simulink model "Multi_drones_deri_and_intro_compare"  (R2021a)
settings: Solver=ode4  StartTime=0.0  StopTime=50  FixedStep=0.005  RelTol=1e-3
(part 2 of 7)

== system Multi_drones_deri_and_intro_compare/Controller 4/High-level system ==
  L : Inport
  info_commu : Inport  Port=2
  bar_delta : Inport  Port=3
  a_d : Inport  Port=4
  Bus Creator : BusCreator  Inputs=3
  Bus Creator1 : BusCreator  Inputs=2
  Controller : MATLAB Function  TreatAsAtomicUnit=on
  Information subtracting : MATLAB Function  TreatAsAtomicUnit=on
  Saturation : Saturate  UpperLimit=0.2  LowerLimit=-0.2
  Virtual sliding variable 4 : Scope
  Virtual tracking error 4 : Scope
  bar_u_i : Scope
  bar_v : Integrator  InitialCondition=[0;0;0]  ContinuousStateAttributes='speed'
  bar_v_i : Scope
  bar_x : Integrator  Tag=Position_x1  InitialCondition=InitialCondition  ContinuousStateAttributes='position'
  bar_x_i : Scope
  new_ref : Outport
  States_virtual : Outport  Port=2
  wires:
  Information subtracting/1(delta_xi) -> Controller/1(delta_xi), Virtual tracking error 4/1
  Information subtracting/4(sat_dot) -> Controller/4(sat_dot)
  info_commu/1 -> Information subtracting/2(info_commu)
  bar_delta/1 -> Information subtracting/3(bar_delta)
  L/1 -> Information subtracting/1(L)
  a_d/1 -> Controller/5(a_di)
  bar_v/1 -> Bus Creator1/2, bar_v_i/1, Bus Creator/2, bar_x/1
  Bus Creator/1 -> new_ref/1
  bar_x/1 -> Bus Creator1/1, Bus Creator/1, bar_x_i/1
  Bus Creator1/1 -> States_virtual/1
  Controller/1(u_i) -> Saturation/1
  Saturation/1 -> bar_u_i/1, Bus Creator/3, bar_v/1
  Information subtracting/2(delta_vi) -> Controller/2(delta_vi)
  Information subtracting/3(s_i) -> Virtual sliding variable 4/1, Controller/3(s_i)

== system Multi_drones_deri_and_intro_compare/Controller 4/Quadcopter model ==
  u_i : Inport
  w_hat_p : Inport  Port=2
  w_hat_a : Inport  Port=3
  Add : Sum  Inputs=+-
  Add1 : Sum  Inputs=+-
  Bus Creator : BusCreator  Inputs=2
  Clock : Clock
  Quadcopter dynamics : MATLAB Function  TreatAsAtomicUnit=on
  f_a : Scope
  f_p : Scope
  quad_v : Scope
  quad_x : Scope
  v_int : Integrator  InitialCondition=[0;0;0;0;0;0]
  w_tilde_a : Scope
  w_tilde_p : Scope
  x_int : Integrator  InitialCondition=InitialCondition
  states_i : Outport
  wires:
  u_i/1 -> Quadcopter dynamics/2(u_i)
  Quadcopter dynamics/1(x_ddot) -> v_int/1
  x_int/1 -> Quadcopter dynamics/1(x_i), quad_x/1, Bus Creator/1
  v_int/1 -> Bus Creator/2, quad_v/1, Quadcopter dynamics/4(v_i), x_int/1
  Bus Creator/1 -> states_i/1
  Quadcopter dynamics/2(w_a) -> Add/1, f_a/1
  w_hat_a/1 -> Add/2
  Add/1 -> w_tilde_a/1
  Clock/1 -> Quadcopter dynamics/3(t)
  Quadcopter dynamics/3(w_p) -> f_p/1, Add1/1
  w_hat_p/1 -> Add1/2
  Add1/1 -> w_tilde_p/1

== system Multi_drones_deri_and_intro_compare/Controller 5/Controller ==
  note: Change the serial number here
  note: Change the serial number here
  note: Change the serial number here
  states_i : Inport
  ref_x_p : Inport  Port=2
  psi_id : Inport  Port=3
  Attitude controller : Subsystem
      settings: PortSchema="{\"entries\":[{\"content\":{\"sides\":[{\"content\":{\"connectorIds\":[\"In1\",\"In2\",\"In3\"]},\"type\":\"ConnectorPlacement.EquallySpacedRectSide\",\"uuid\":\"fa62b1eb-ed3d-4a84-b897-b51f17bb9d42\"},{\"content\":{\"connectorIds\":[\"Out1\"],\"side\":\"RIGHT\"},\"type\":\"ConnectorPlacement.EquallySpacedRectSide\",\"uuid\":\"9b6b7a3c-e484-45bf-bd32-fe40ffeb0d28\"},{\"content\":{\"connectorIds\":[\"Out2\"],\"side\":\"TOP\"},\"type\":\"ConnectorPlacement.EquallySpacedRectSide\",\"uuid\":\"d1ffdbb9-18c9-4f2c-95a6-bf4c2ab27347\"}]},\"type\":\"ConnectorPlacement.EquallySpacedConnector\",\"uuid\":\"2804a1df-60db-43d6-95d2-4687dde4bd06\"}],\"packageUris\":[\"http://schema.mathworks.com/mf0/Connector/R2020b\"],\"version\":\"1.0\"}"
  Constant : Constant  Value=13.72  VectorParams1D=off
  Manual Switch : ManualSwitch
  Nominal control calculation : MATLAB Function  TreatAsAtomicUnit=on
  Position controller1 : Subsystem
      settings: PortSchema="{\"entries\":[{\"content\":{\"sides\":[{\"content\":{\"connectorIds\":[\"In1\",\"In2\",\"In3\"]},\"type\":\"ConnectorPlacement.EquallySpacedRectSide\",\"uuid\":\"6f6db54a-065c-4c68-96d3-ce6f9528f7c2\"},{\"content\":{\"connectorIds\":[\"Out1\"],\"side\":\"RIGHT\"},\"type\":\"ConnectorPlacement.EquallySpacedRectSide\",\"uuid\":\"eab021de-0481-49e0-8239-dbc5993eb5fa\"},{\"content\":{\"connectorIds\":[\"Out2\"],\"side\":\"TOP\"},\"type\":\"ConnectorPlacement.EquallySpacedRectSide\",\"uuid\":\"c7d044cf-1b8b-40e5-8601-940ebebd0ccb\"},{\"content\":{\"connectorIds\":[],\"side\":\"BOTTOM\"},\"type\":\"ConnectorPlacement.EquallySpacedRectSide\",\"uuid\":\"6c5daa93-b438-4c34-9741-3ab1f6346320\"}]},\"type\":\"ConnectorPlacement.EquallySpacedConnector\",\"uuid\":\"bb7db914-9823-41d6-a8ba-39b4d2976335\"}],\"packageUris\":[\"http://schema.mathworks.com/mf0/Connector/R2020b\"],\"version\":\"1.0\"}"
  Real control input : MATLAB Function  TreatAsAtomicUnit=on
  Reverse calculation : Subsystem
      settings: PortSchema="{\"entries\":[{\"content\":{\"sides\":[{\"content\":{\"connectorIds\":[\"In1\",\"In2\"]},\"type\":\"ConnectorPlacement.EquallySpacedRectSide\",\"uuid\":\"a324fb00-881d-40c1-b7da-a9c7871d46ce\"},{\"content\":{\"connectorIds\":[\"Out1\",\"Out2\"],\"side\":\"RIGHT\"},\"type\":\"ConnectorPlacement.EquallySpacedRectSide\",\"uuid\":\"58739d0b-b2b3-44e8-8796-6553ce8d5a15\"},{\"content\":{\"connectorIds\":[\"In3\"],\"side\":\"TOP\"},\"type\":\"ConnectorPlacement.EquallySpacedRectSide\",\"uuid\":\"8c9acd48-a842-4889-b739-8799f04ac800\"}]},\"type\":\"ConnectorPlacement.EquallySpacedConnector\",\"uuid\":\"9c847f57-6425-42e5-8be7-b64809e08636\"}],\"packageUris\":[\"http://schema.mathworks.com/mf0/Connector/R2020b\"],\"version\":\"1.0\"}"
  Scope : Scope
  T_id : Scope
  atti_ref : Scope
  u : Scope
  u_ip : Scope
  u_nom_a : Scope
  u_nom_p : Scope
  u_i : Outport
  w_hat_p : Outport  Port=2
  w_hat_a : Outport  Port=3
  wires:
  Attitude controller/1(u_I_a) -> Real control input/1(u_i_a)
  ref_x_p/1 -> Position controller1/2(ref_x_p)
  states_i/1 -> Position controller1/1(states_i), Reverse calculation/3(states_i), Attitude controller/1(states_i), Nominal control calculation/1(states_i)
  Nominal control calculation/1(u_nom_p) -> Position controller1/3(u_nom_p), u_nom_p/1
  Nominal control calculation/2(u_nom_a) -> Attitude controller/3(u_nom_a), u_nom_a/1
  Position controller1/1(u_i_p) -> Reverse calculation/2(u_ip), u_ip/1
  Reverse calculation/1(atti_ref) -> Attitude controller/2(atti_ref), atti_ref/1
  Position controller1/2(w_hat_p) -> w_hat_p/1
  Attitude controller/2(w_hat_a) -> w_hat_a/1
  Constant/1 -> Manual Switch/2
  Reverse calculation/2(T_i_d) -> Manual Switch/1
  Manual Switch/1 -> T_id/1, Real control input/2(T_id)
  Real control input/2(u_i) -> Nominal control calculation/2(u_i), u/1, u_i/1
  Real control input/1(tau_i) -> Scope/1
  psi_id/1 -> Reverse calculation/1(psi_id)

== system Multi_drones_deri_and_intro_compare/Controller 5/High-level system ==
  L : Inport
  info_commu : Inport  Port=2
  bar_delta : Inport  Port=3
  a_d : Inport  Port=4
  Bus Creator : BusCreator  Inputs=3
  Bus Creator1 : BusCreator  Inputs=2
  Controller : MATLAB Function  TreatAsAtomicUnit=on
  Information subtracting : MATLAB Function  TreatAsAtomicUnit=on
  Saturation : Saturate  UpperLimit=0.2  LowerLimit=-0.2
  Virtual sliding variable 5 : Scope
  Virtual tracking error 5 : Scope
  bar_u_i : Scope
  bar_v : Integrator  InitialCondition=[0;0;0]  ContinuousStateAttributes='speed'
  bar_v_i : Scope
  bar_x : Integrator  Tag=Position_x1  InitialCondition=InitialCondition  ContinuousStateAttributes='position'
  bar_x_i : Scope
  new_ref : Outport
  States_virtual : Outport  Port=2
  wires:
  Information subtracting/1(delta_xi) -> Controller/1(delta_xi), Virtual tracking error 5/1
  Information subtracting/4(sat_dot) -> Controller/4(sat_dot)
  info_commu/1 -> Information subtracting/2(info_commu)
  bar_delta/1 -> Information subtracting/3(bar_delta)
  L/1 -> Information subtracting/1(L)
  a_d/1 -> Controller/5(a_di)
  bar_v/1 -> Bus Creator1/2, bar_v_i/1, Bus Creator/2, bar_x/1
  Bus Creator/1 -> new_ref/1
  bar_x/1 -> Bus Creator1/1, Bus Creator/1, bar_x_i/1
  Bus Creator1/1 -> States_virtual/1
  Controller/1(u_i) -> Saturation/1
  Saturation/1 -> bar_u_i/1, Bus Creator/3, bar_v/1
  Information subtracting/2(delta_vi) -> Controller/2(delta_vi)
  Information subtracting/3(s_i) -> Virtual sliding variable 5/1, Controller/3(s_i)

== system Multi_drones_deri_and_intro_compare/Controller 5/Quadcopter model ==
  u_i : Inport
  w_hat_p : Inport  Port=2
  w_hat_a : Inport  Port=3
  Add : Sum  Inputs=+-
  Add1 : Sum  Inputs=+-
  Bus Creator : BusCreator  Inputs=2
  Clock : Clock
  Quadcopter dynamics : MATLAB Function  TreatAsAtomicUnit=on
  f_a : Scope
  f_p : Scope
  quad_v : Scope
  quad_x : Scope
  v_int : Integrator  InitialCondition=[0;0;0;0;0;0]
  w_tilde_a : Scope
  w_tilde_p : Scope
  x_int : Integrator  InitialCondition=InitialCondition
  states_i : Outport
  wires:
  u_i/1 -> Quadcopter dynamics/2(u_i)
  Quadcopter dynamics/1(x_ddot) -> v_int/1
  x_int/1 -> Quadcopter dynamics/1(x_i), quad_x/1, Bus Creator/1
  v_int/1 -> Bus Creator/2, quad_v/1, Quadcopter dynamics/4(v_i), x_int/1
  Bus Creator/1 -> states_i/1
  Quadcopter dynamics/2(w_a) -> Add/1, f_a/1
  w_hat_a/1 -> Add/2
  Add/1 -> w_tilde_a/1
  Clock/1 -> Quadcopter dynamics/3(t)
  Quadcopter dynamics/3(w_p) -> f_p/1, Add1/1
  w_hat_p/1 -> Add1/2
  Add1/1 -> w_tilde_p/1

== system Multi_drones_deri_and_intro_compare/Controller 6/Controller ==
  note: Change the serial number here
  note: Change the serial number here
  note: Change the serial number here
  states_i : Inport
  ref_x_p : Inport  Port=2
  psi_id : Inport  Port=3
  Attitude controller : Subsystem
      settings: PortSchema="{\"entries\":[{\"content\":{\"sides\":[{\"content\":{\"connectorIds\":[\"In1\",\"In2\",\"In3\"]},\"type\":\"ConnectorPlacement.EquallySpacedRectSide\",\"uuid\":\"fa62b1eb-ed3d-4a84-b897-b51f17bb9d42\"},{\"content\":{\"connectorIds\":[\"Out1\"],\"side\":\"RIGHT\"},\"type\":\"ConnectorPlacement.EquallySpacedRectSide\",\"uuid\":\"9b6b7a3c-e484-45bf-bd32-fe40ffeb0d28\"},{\"content\":{\"connectorIds\":[\"Out2\"],\"side\":\"TOP\"},\"type\":\"ConnectorPlacement.EquallySpacedRectSide\",\"uuid\":\"d1ffdbb9-18c9-4f2c-95a6-bf4c2ab27347\"}]},\"type\":\"ConnectorPlacement.EquallySpacedConnector\",\"uuid\":\"2804a1df-60db-43d6-95d2-4687dde4bd06\"}],\"packageUris\":[\"http://schema.mathworks.com/mf0/Connector/R2020b\"],\"version\":\"1.0\"}"
  Constant : Constant  Value=13.72  VectorParams1D=off
  Manual Switch : ManualSwitch
  Nominal control calculation : MATLAB Function  TreatAsAtomicUnit=on
  Position controller1 : Subsystem
      settings: PortSchema="{\"entries\":[{\"content\":{\"sides\":[{\"content\":{\"connectorIds\":[\"In1\",\"In2\",\"In3\"]},\"type\":\"ConnectorPlacement.EquallySpacedRectSide\",\"uuid\":\"6f6db54a-065c-4c68-96d3-ce6f9528f7c2\"},{\"content\":{\"connectorIds\":[\"Out1\"],\"side\":\"RIGHT\"},\"type\":\"ConnectorPlacement.EquallySpacedRectSide\",\"uuid\":\"eab021de-0481-49e0-8239-dbc5993eb5fa\"},{\"content\":{\"connectorIds\":[\"Out2\"],\"side\":\"TOP\"},\"type\":\"ConnectorPlacement.EquallySpacedRectSide\",\"uuid\":\"c7d044cf-1b8b-40e5-8601-940ebebd0ccb\"},{\"content\":{\"connectorIds\":[],\"side\":\"BOTTOM\"},\"type\":\"ConnectorPlacement.EquallySpacedRectSide\",\"uuid\":\"6c5daa93-b438-4c34-9741-3ab1f6346320\"}]},\"type\":\"ConnectorPlacement.EquallySpacedConnector\",\"uuid\":\"bb7db914-9823-41d6-a8ba-39b4d2976335\"}],\"packageUris\":[\"http://schema.mathworks.com/mf0/Connector/R2020b\"],\"version\":\"1.0\"}"
  Real control input : MATLAB Function  TreatAsAtomicUnit=on
  Reverse calculation : Subsystem
      settings: PortSchema="{\"entries\":[{\"content\":{\"sides\":[{\"content\":{\"connectorIds\":[\"In1\",\"In2\"]},\"type\":\"ConnectorPlacement.EquallySpacedRectSide\",\"uuid\":\"a324fb00-881d-40c1-b7da-a9c7871d46ce\"},{\"content\":{\"connectorIds\":[\"Out1\",\"Out2\"],\"side\":\"RIGHT\"},\"type\":\"ConnectorPlacement.EquallySpacedRectSide\",\"uuid\":\"58739d0b-b2b3-44e8-8796-6553ce8d5a15\"},{\"content\":{\"connectorIds\":[\"In3\"],\"side\":\"TOP\"},\"type\":\"ConnectorPlacement.EquallySpacedRectSide\",\"uuid\":\"8c9acd48-a842-4889-b739-8799f04ac800\"}]},\"type\":\"ConnectorPlacement.EquallySpacedConnector\",\"uuid\":\"9c847f57-6425-42e5-8be7-b64809e08636\"}],\"packageUris\":[\"http://schema.mathworks.com/mf0/Connector/R2020b\"],\"version\":\"1.0\"}"
  Scope : Scope
  T_id : Scope
  atti_ref : Scope
  u : Scope
  u_ip : Scope
  u_nom_a : Scope
  u_nom_p : Scope
  u_i : Outport
  w_hat_p : Outport  Port=2
  w_hat_a : Outport  Port=3
  wires:
  Attitude controller/1(u_I_a) -> Real control input/1(u_i_a)
  ref_x_p/1 -> Position controller1/2(ref_x_p)
  states_i/1 -> Position controller1/1(states_i), Reverse calculation/3(states_i), Attitude controller/1(states_i), Nominal control calculation/1(states_i)
  Nominal control calculation/1(u_nom_p) -> Position controller1/3(u_nom_p), u_nom_p/1
  Nominal control calculation/2(u_nom_a) -> Attitude controller/3(u_nom_a), u_nom_a/1
  Position controller1/1(u_i_p) -> Reverse calculation/2(u_ip), u_ip/1
  Reverse calculation/1(atti_ref) -> Attitude controller/2(atti_ref), atti_ref/1
  Position controller1/2(w_hat_p) -> w_hat_p/1
  Attitude controller/2(w_hat_a) -> w_hat_a/1
  Constant/1 -> Manual Switch/2
  Reverse calculation/2(T_i_d) -> Manual Switch/1
  Manual Switch/1 -> T_id/1, Real control input/2(T_id)
  Real control input/2(u_i) -> Nominal control calculation/2(u_i), u/1, u_i/1
  Real control input/1(tau_i) -> Scope/1
  psi_id/1 -> Reverse calculation/1(psi_id)

== system Multi_drones_deri_and_intro_compare/Controller 6/High-level system ==
  L : Inport
  info_commu : Inport  Port=2
  bar_delta : Inport  Port=3
  a_d : Inport  Port=4
  Bus Creator : BusCreator  Inputs=3
  Bus Creator1 : BusCreator  Inputs=2
  Controller : MATLAB Function  TreatAsAtomicUnit=on
  Information subtracting : MATLAB Function  TreatAsAtomicUnit=on
  Saturation : Saturate  UpperLimit=0.2  LowerLimit=-0.2
  Virtual sliding variable : Scope
  Virtual tracking error : Scope
  bar_u_i : Scope
  bar_v : Integrator  InitialCondition=[0;0;0]  ContinuousStateAttributes='speed'
  bar_v_i : Scope
  bar_x : Integrator  Tag=Position_x1  InitialCondition=InitialCondition  ContinuousStateAttributes='position'
  bar_x_i : Scope
  new_ref : Outport
  States_virtual : Outport  Port=2
  wires:
  Information subtracting/1(delta_xi) -> Controller/1(delta_xi), Virtual tracking error/1
  Information subtracting/4(sat_dot) -> Controller/4(sat_dot)
  info_commu/1 -> Information subtracting/2(info_commu)
  bar_delta/1 -> Information subtracting/3(bar_delta)
  L/1 -> Information subtracting/1(L)
  a_d/1 -> Controller/5(a_di)
  bar_v/1 -> Bus Creator1/2, bar_v_i/1, Bus Creator/2, bar_x/1
  Bus Creator/1 -> new_ref/1
  bar_x/1 -> Bus Creator1/1, Bus Creator/1, bar_x_i/1
  Bus Creator1/1 -> States_virtual/1
  Controller/1(u_i) -> Saturation/1
  Saturation/1 -> bar_u_i/1, Bus Creator/3, bar_v/1
  Information subtracting/2(delta_vi) -> Controller/2(delta_vi)
  Information subtracting/3(s_i) -> Virtual sliding variable/1, Controller/3(s_i)

== system Multi_drones_deri_and_intro_compare/Controller 6/Quadcopter model ==
  u_i : Inport
  w_hat_p : Inport  Port=2
  w_hat_a : Inport  Port=3
  Add : Sum  Inputs=+-
  Add1 : Sum  Inputs=+-
  Bus Creator : BusCreator  Inputs=2
  Clock : Clock
  Quadcopter dynamics : MATLAB Function  TreatAsAtomicUnit=on
  f_a : Scope
  f_p : Scope
  quad_v : Scope
  quad_x : Scope
  v_int : Integrator  InitialCondition=[0;0;0;0;0;0]
  w_tilde_a : Scope
  w_tilde_p : Scope
  x_int : Integrator  InitialCondition=InitialCondition
  states_i : Outport
  wires:
  u_i/1 -> Quadcopter dynamics/2(u_i)
  Quadcopter dynamics/1(x_ddot) -> v_int/1
  x_int/1 -> Quadcopter dynamics/1(x_i), quad_x/1, Bus Creator/1
  v_int/1 -> Bus Creator/2, quad_v/1, Quadcopter dynamics/4(v_i), x_int/1
  Bus Creator/1 -> states_i/1
  Quadcopter dynamics/2(w_a) -> Add/1, f_a/1
  w_hat_a/1 -> Add/2
  Add/1 -> w_tilde_a/1
  Clock/1 -> Quadcopter dynamics/3(t)
  Quadcopter dynamics/3(w_p) -> f_p/1, Add1/1
  w_hat_p/1 -> Add1/2
  Add1/1 -> w_tilde_p/1

== system Multi_drones_deri_and_intro_compare/Reference generator/Coordinate reference ==
  Time : Inport
  Ref_gene : MATLAB Function  TreatAsAtomicUnit=on
  x_d_p : Outport
  v_d_p : Outport  Port=2
  a_d_p : Outport  Port=3
  wires:
  Time/1 -> Ref_gene/1(t)
  Ref_gene/1(x_d_p) -> x_d_p/1
  Ref_gene/2(v_d_p) -> v_d_p/1
  Ref_gene/3(a_d_p) -> a_d_p/1

== system Multi_drones_deri_and_intro_compare/Controller 1/Controller/Attitude controller ==
  states_i : Inport
  atti_ref : Inport  Port=2
  u_nom_a : Inport  Port=3
  Angle controller : MATLAB Function  TreatAsAtomicUnit=on
  Angle error : MATLAB Function  TreatAsAtomicUnit=on
  Angle sliding variable : MATLAB Function  TreatAsAtomicUnit=on
  Attitude loop observer : Subsystem
      settings: PortSchema="{\"entries\":[{\"content\":{\"sides\":[{\"content\":{\"connectorIds\":[\"In1\",\"In2\",\"In3\"]},\"type\":\"ConnectorPlacement.EquallySpacedRectSide\",\"uuid\":\"edf82c9f-eb15-4775-9311-d50d92fa47fd\"},{\"content\":{\"connectorIds\":[\"Out1\",\"Out2\"],\"side\":\"RIGHT\"},\"type\":\"ConnectorPlacement.EquallySpacedRectSide\",\"uuid\":\"b90416f6-8117-4ec7-8f9a-c5fae9711eab\"},{\"content\":{\"connectorIds\":[\"In4\"],\"side\":\"TOP\"},\"type\":\"ConnectorPlacement.EquallySpacedRectSide\",\"uuid\":\"e7e2e1a9-76d3-420a-917d-b73182cbe298\"}]},\"type\":\"ConnectorPlacement.EquallySpacedConnector\",\"uuid\":\"4fc8298e-c3da-4bdd-b1ba-c07bafbec956\"}],\"packageUris\":[\"http://schema.mathworks.com/mf0/Connector/R2020b\"],\"version\":\"1.0\"}"
  Scope : Scope
  Sliding mode differentiator : Subsystem
      settings: PortSchema="{\"entries\":[{\"content\":{\"sides\":[{\"content\":{\"connectorIds\":[\"In1\"]},\"type\":\"ConnectorPlacement.EquallySpacedRectSide\",\"uuid\":\"d0355641-aeac-4820-b7cd-f9621efbd127\"},{\"content\":{\"connectorIds\":[\"Out1\",\"Out2\"],\"side\":\"RIGHT\"},\"type\":\"ConnectorPlacement.EquallySpacedRectSide\",\"uuid\":\"185ec072-6206-4946-bebc-a6564ad10b6f\"},{\"content\":{\"connectorIds\":[\"Out3\"],\"side\":\"TOP\"},\"type\":\"ConnectorPlacement.EquallySpacedRectSide\",\"uuid\":\"43c1499b-0abd-4d60-8d0e-f99edfc99abb\"}]},\"type\":\"ConnectorPlacement.EquallySpacedConnector\",\"uuid\":\"7137f0d1-a693-433d-9f21-56f33280b1ef\"}],\"packageUris\":[\"http://schema.mathworks.com/mf0/Connector/R2020b\"],\"version\":\"1.0\"}"
  State selection : MATLAB Function  TreatAsAtomicUnit=on
  delta_v_a : Scope
  delta_x_a_1 : Scope
  s_i_a_1 : Scope
  u_I_a : Outport
  w_hat_a : Outport  Port=2
  wires:
  Angle controller/1(u_i_a) -> Scope/1, u_I_a/1
  Angle sliding variable/1(s_i_a) -> s_i_a_1/1, Angle controller/2(s_i_a)
  atti_ref/1 -> Sliding mode differentiator/1(Reference)
  states_i/1 -> State selection/1(states_i), Attitude loop observer/1(states_i)
  State selection/1(x_i_a) -> Attitude loop observer/2(x_i_a), Angle error/1(x_i_a)
  State selection/2(v_i_a) -> Attitude loop observer/3(v_i_a), Angle error/2(v_i_a)
  Sliding mode differentiator/3(ang_d) -> Angle error/3(ang_d)
  Angle error/1(delta_x_a) -> delta_x_a_1/1, Angle sliding variable/1(delta_x_a), Angle controller/3(delta_x_a)
  Angle error/2(delta_v_a) -> delta_v_a/1, Angle controller/4(delta_v_a), Angle sliding variable/2(delta_v_a)
  Attitude loop observer/2(w_hat_a) -> Angle controller/1(w_hat_a)
  Sliding mode differentiator/2(ang_d_ddot) -> Angle controller/5(ang_d_ddot)
  u_nom_a/1 -> Attitude loop observer/4(u_nom_a)
  Sliding mode differentiator/1(ang_d_dot) -> Angle error/4(ang_d_dot)
  Attitude loop observer/1(w_hat_a_actual) -> w_hat_a/1

== system Multi_drones_deri_and_intro_compare/Controller 1/Controller/Position controller1 ==
  note: Note that a saturation is added here
  states_i : Inport
  ref_x_p : Inport  Port=2
  u_nom_p : Inport  Port=3
  Constant : Constant  Value=[0;0;0]  VectorParams1D=off
  Error calculation : MATLAB Function  TreatAsAtomicUnit=on
  Position loop observer : Subsystem  mask{InitialCondition=[4;1;0]}
      mask prompts: InitialCondition "Simulink:blkprm_prompts:IntegratorInitCond"
      settings: PortSchema="{\"entries\":[{\"content\":{\"sides\":[{\"content\":{\"connectorIds\":[\"In1\",\"In2\",\"In3\"]},\"type\":\"ConnectorPlacement.EquallySpacedRectSide\",\"uuid\":\"edf82c9f-eb15-4775-9311-d50d92fa47fd\"},{\"content\":{\"connectorIds\":[\"Out1\",\"Out2\"],\"side\":\"RIGHT\"},\"type\":\"ConnectorPlacement.EquallySpacedRectSide\",\"uuid\":\"b90416f6-8117-4ec7-8f9a-c5fae9711eab\"},{\"content\":{\"connectorIds\":[\"In4\"],\"side\":\"TOP\"},\"type\":\"ConnectorPlacement.EquallySpacedRectSide\",\"uuid\":\"e7e2e1a9-76d3-420a-917d-b73182cbe298\"}]},\"type\":\"ConnectorPlacement.EquallySpacedConnector\",\"uuid\":\"4fc8298e-c3da-4bdd-b1ba-c07bafbec956\"}],\"packageUris\":[\"http://schema.mathworks.com/mf0/Connector/R2020b\"],\"version\":\"1.0\"}"
      mask TypeOptions InitialCondition: Integrator1/InitialCondition
      mask DialogControl InitialCondition Prompt: Initial condition:
  Reference selection (Low) : MATLAB Function  TreatAsAtomicUnit=on
  State selection : MATLAB Function  TreatAsAtomicUnit=on
  Virtual position controller : MATLAB Function  TreatAsAtomicUnit=on
  delta_v_p : Scope
  delta_x_p_1 : Scope
  s_i_p_1 : Scope
  u_i : Scope
  u_i_p : Outport
  w_hat_p : Outport  Port=2
  wires:
  states_i/1 -> Position loop observer/1(states_i), State selection/1(states_i)
  ref_x_p/1 -> Reference selection (Low)/1(ref_x_p)
  Reference selection (Low)/1(x_i_p_d) -> Error calculation/4(x_i_p_d)
  Reference selection (Low)/2(v_i_p_d) -> Error calculation/5(v_i_p_d)
  State selection/2(v_i_p) -> Position loop observer/3(v_i_p), Error calculation/2(v_i_p)
  State selection/1(x_i_p) -> Position loop observer/2(x_i_p), Error calculation/1(x_i_p)
  u_nom_p/1 -> Position loop observer/4(u_nom_p)
  Reference selection (Low)/3(a_i_p_d) -> Virtual position controller/5(a_i_p_d)
  Constant/1 -> Error calculation/3(Phi_i)
  Error calculation/3(delta_v_p) -> delta_v_p/1, Virtual position controller/4(delta_v_p)
  Error calculation/2(delta_x_p) -> delta_x_p_1/1, Virtual position controller/3(delta_x_p)
  Error calculation/1(s_i_p) -> s_i_p_1/1, Virtual position controller/2(s_i_p)
  Virtual position controller/1(u_i_p) -> u_i_p/1, u_i/1
  Position loop observer/1(w_hat_p_actual) -> w_hat_p/1
  Position loop observer/2(w_hat_p) -> Virtual position controller/1(w_hat_p)

== system Multi_drones_deri_and_intro_compare/Controller 1/Controller/Reverse calculation ==
  psi_id : Inport
  u_ip : Inport  Port=2
  states_i : Inport  Port=3
  Reverse calculation : MATLAB Function  TreatAsAtomicUnit=on
  State selection : MATLAB Function  TreatAsAtomicUnit=on
  atti_ref : Outport
  T_i_d : Outport  Port=2
  wires:
  Reverse calculation/2(T_i_d) -> T_i_d/1
  Reverse calculation/1(atti_ref) -> atti_ref/1
  states_i/1 -> State selection/1(states_i)
  State selection/1(x_i_a) -> Reverse calculation/3(x_i_a)
  u_ip/1 -> Reverse calculation/2(u_i_p)
  psi_id/1 -> Reverse calculation/1(psi_i_d)

== system Multi_drones_deri_and_intro_compare/Controller 2/Controller/Attitude controller ==
  states_i : Inport
  atti_ref : Inport  Port=2
  u_nom_a : Inport  Port=3
  Angle controller : MATLAB Function  TreatAsAtomicUnit=on
  Angle error : MATLAB Function  TreatAsAtomicUnit=on
  Angle sliding variable : MATLAB Function  TreatAsAtomicUnit=on
  Attitude loop observer : Subsystem
      settings: PortSchema="{\"entries\":[{\"content\":{\"sides\":[{\"content\":{\"connectorIds\":[\"In1\",\"In2\",\"In3\"]},\"type\":\"ConnectorPlacement.EquallySpacedRectSide\",\"uuid\":\"edf82c9f-eb15-4775-9311-d50d92fa47fd\"},{\"content\":{\"connectorIds\":[\"Out1\",\"Out2\"],\"side\":\"RIGHT\"},\"type\":\"ConnectorPlacement.EquallySpacedRectSide\",\"uuid\":\"b90416f6-8117-4ec7-8f9a-c5fae9711eab\"},{\"content\":{\"connectorIds\":[\"In4\"],\"side\":\"TOP\"},\"type\":\"ConnectorPlacement.EquallySpacedRectSide\",\"uuid\":\"e7e2e1a9-76d3-420a-917d-b73182cbe298\"}]},\"type\":\"ConnectorPlacement.EquallySpacedConnector\",\"uuid\":\"4fc8298e-c3da-4bdd-b1ba-c07bafbec956\"}],\"packageUris\":[\"http://schema.mathworks.com/mf0/Connector/R2020b\"],\"version\":\"1.0\"}"
  Scope : Scope
  Sliding mode differentiator : Subsystem
      settings: PortSchema="{\"entries\":[{\"content\":{\"sides\":[{\"content\":{\"connectorIds\":[\"In1\"]},\"type\":\"ConnectorPlacement.EquallySpacedRectSide\",\"uuid\":\"d0355641-aeac-4820-b7cd-f9621efbd127\"},{\"content\":{\"connectorIds\":[\"Out1\",\"Out2\"],\"side\":\"RIGHT\"},\"type\":\"ConnectorPlacement.EquallySpacedRectSide\",\"uuid\":\"185ec072-6206-4946-bebc-a6564ad10b6f\"},{\"content\":{\"connectorIds\":[\"Out3\"],\"side\":\"TOP\"},\"type\":\"ConnectorPlacement.EquallySpacedRectSide\",\"uuid\":\"43c1499b-0abd-4d60-8d0e-f99edfc99abb\"}]},\"type\":\"ConnectorPlacement.EquallySpacedConnector\",\"uuid\":\"7137f0d1-a693-433d-9f21-56f33280b1ef\"}],\"packageUris\":[\"http://schema.mathworks.com/mf0/Connector/R2020b\"],\"version\":\"1.0\"}"
  State selection : MATLAB Function  TreatAsAtomicUnit=on
  delta_v_a : Scope
  delta_x_a_2 : Scope
  s_i_a_2 : Scope
  u_I_a : Outport
  w_hat_a : Outport  Port=2
  wires:
  Angle controller/1(u_i_a) -> Scope/1, u_I_a/1
  Angle sliding variable/1(s_i_a) -> s_i_a_2/1, Angle controller/2(s_i_a)
  atti_ref/1 -> Sliding mode differentiator/1(Reference)
  states_i/1 -> State selection/1(states_i), Attitude loop observer/1(states_i)
  State selection/1(x_i_a) -> Attitude loop observer/2(x_i_a), Angle error/1(x_i_a)
  State selection/2(v_i_a) -> Attitude loop observer/3(v_i_a), Angle error/2(v_i_a)
  Sliding mode differentiator/3(ang_d) -> Angle error/3(ang_d)
  Angle error/1(delta_x_a) -> delta_x_a_2/1, Angle sliding variable/1(delta_x_a), Angle controller/3(delta_x_a)
  Angle error/2(delta_v_a) -> delta_v_a/1, Angle controller/4(delta_v_a), Angle sliding variable/2(delta_v_a)
  Attitude loop observer/2(w_hat_a) -> Angle controller/1(w_hat_a)
  Sliding mode differentiator/2(ang_d_ddot) -> Angle controller/5(ang_d_ddot)
  u_nom_a/1 -> Attitude loop observer/4(u_nom_a)
  Sliding mode differentiator/1(ang_d_dot) -> Angle error/4(ang_d_dot)
  Attitude loop observer/1(w_hat_a_actual) -> w_hat_a/1

== system Multi_drones_deri_and_intro_compare/Controller 2/Controller/Position controller1 ==
  note: Note that a saturation is added here
  states_i : Inport
  ref_x_p : Inport  Port=2
  u_nom_p : Inport  Port=3
  Constant : Constant  Value=[0;0;0]  VectorParams1D=off
  Error calculation : MATLAB Function  TreatAsAtomicUnit=on
  Position loop observer : Subsystem  mask{InitialCondition=[1;2;0]}
      mask prompts: InitialCondition "Simulink:blkprm_prompts:IntegratorInitCond"
      settings: PortSchema="{\"entries\":[{\"content\":{\"sides\":[{\"content\":{\"connectorIds\":[\"In1\",\"In2\",\"In3\"]},\"type\":\"ConnectorPlacement.EquallySpacedRectSide\",\"uuid\":\"edf82c9f-eb15-4775-9311-d50d92fa47fd\"},{\"content\":{\"connectorIds\":[\"Out1\",\"Out2\"],\"side\":\"RIGHT\"},\"type\":\"ConnectorPlacement.EquallySpacedRectSide\",\"uuid\":\"b90416f6-8117-4ec7-8f9a-c5fae9711eab\"},{\"content\":{\"connectorIds\":[\"In4\"],\"side\":\"TOP\"},\"type\":\"ConnectorPlacement.EquallySpacedRectSide\",\"uuid\":\"e7e2e1a9-76d3-420a-917d-b73182cbe298\"}]},\"type\":\"ConnectorPlacement.EquallySpacedConnector\",\"uuid\":\"4fc8298e-c3da-4bdd-b1ba-c07bafbec956\"}],\"packageUris\":[\"http://schema.mathworks.com/mf0/Connector/R2020b\"],\"version\":\"1.0\"}"
      mask TypeOptions InitialCondition: x_int/InitialCondition
      mask DialogControl InitialCondition Prompt: Initial condition:
  Reference selection (Low) : MATLAB Function  TreatAsAtomicUnit=on
  State selection : MATLAB Function  TreatAsAtomicUnit=on
  Virtual position controller : MATLAB Function  TreatAsAtomicUnit=on
  delta_v_p_2 : Scope
  delta_x_p_2 : Scope
  s_i_p_2 : Scope
  u_i : Scope
  u_i_p : Outport
  w_hat_p : Outport  Port=2
  wires:
  states_i/1 -> Position loop observer/1(states_i), State selection/1(states_i)
  ref_x_p/1 -> Reference selection (Low)/1(ref_x_p)
  Reference selection (Low)/1(x_i_p_d) -> Error calculation/4(x_i_p_d)
  Reference selection (Low)/2(v_i_p_d) -> Error calculation/5(v_i_p_d)
  State selection/2(v_i_p) -> Position loop observer/3(v_i_p), Error calculation/2(v_i_p)
  State selection/1(x_i_p) -> Position loop observer/2(x_i_p), Error calculation/1(x_i_p)
  u_nom_p/1 -> Position loop observer/4(u_nom_p)
  Position loop observer/2(w_hat_p) -> Virtual position controller/1(w_hat_p)
  Reference selection (Low)/3(a_i_p_d) -> Virtual position controller/5(a_i_p_d)
  Constant/1 -> Error calculation/3(Phi_i)
  Error calculation/3(delta_v_p) -> delta_v_p_2/1, Virtual position controller/4(delta_v_p)
  Error calculation/2(delta_x_p) -> delta_x_p_2/1, Virtual position controller/3(delta_x_p)
  Error calculation/1(s_i_p) -> s_i_p_2/1, Virtual position controller/2(s_i_p)
  Virtual position controller/1(u_i_p) -> u_i_p/1, u_i/1
  Position loop observer/1(w_hat_p_actual) -> w_hat_p/1

== system Multi_drones_deri_and_intro_compare/Controller 2/Controller/Reverse calculation ==
  psi_id : Inport
  u_ip : Inport  Port=2
  states_i : Inport  Port=3
  Reverse calculation : MATLAB Function  TreatAsAtomicUnit=on
  State selection : MATLAB Function  TreatAsAtomicUnit=on
  atti_ref : Outport
  T_i_d : Outport  Port=2
  wires:
  Reverse calculation/2(T_i_d) -> T_i_d/1
  Reverse calculation/1(atti_ref) -> atti_ref/1
  states_i/1 -> State selection/1(states_i)
  State selection/1(x_i_a) -> Reverse calculation/3(x_i_a)
  u_ip/1 -> Reverse calculation/2(u_i_p)
  psi_id/1 -> Reverse calculation/1(psi_i_d)

== system Multi_drones_deri_and_intro_compare/Controller 3/Controller/Attitude controller ==
  states_i : Inport
  atti_ref : Inport  Port=2
  u_nom_a : Inport  Port=3
  Angle controller : MATLAB Function  TreatAsAtomicUnit=on
  Angle error : MATLAB Function  TreatAsAtomicUnit=on
  Angle sliding variable : MATLAB Function  TreatAsAtomicUnit=on
  Attitude loop observer : Subsystem
      settings: PortSchema="{\"entries\":[{\"content\":{\"sides\":[{\"content\":{\"connectorIds\":[\"In1\",\"In2\",\"In3\"]},\"type\":\"ConnectorPlacement.EquallySpacedRectSide\",\"uuid\":\"edf82c9f-eb15-4775-9311-d50d92fa47fd\"},{\"content\":{\"connectorIds\":[\"Out1\",\"Out2\"],\"side\":\"RIGHT\"},\"type\":\"ConnectorPlacement.EquallySpacedRectSide\",\"uuid\":\"b90416f6-8117-4ec7-8f9a-c5fae9711eab\"},{\"content\":{\"connectorIds\":[\"In4\"],\"side\":\"TOP\"},\"type\":\"ConnectorPlacement.EquallySpacedRectSide\",\"uuid\":\"e7e2e1a9-76d3-420a-917d-b73182cbe298\"}]},\"type\":\"ConnectorPlacement.EquallySpacedConnector\",\"uuid\":\"4fc8298e-c3da-4bdd-b1ba-c07bafbec956\"}],\"packageUris\":[\"http://schema.mathworks.com/mf0/Connector/R2020b\"],\"version\":\"1.0\"}"
  Scope : Scope
  Sliding mode differentiator : Subsystem
      settings: PortSchema="{\"entries\":[{\"content\":{\"sides\":[{\"content\":{\"connectorIds\":[\"In1\"]},\"type\":\"ConnectorPlacement.EquallySpacedRectSide\",\"uuid\":\"d0355641-aeac-4820-b7cd-f9621efbd127\"},{\"content\":{\"connectorIds\":[\"Out1\",\"Out2\"],\"side\":\"RIGHT\"},\"type\":\"ConnectorPlacement.EquallySpacedRectSide\",\"uuid\":\"185ec072-6206-4946-bebc-a6564ad10b6f\"},{\"content\":{\"connectorIds\":[\"Out3\"],\"side\":\"TOP\"},\"type\":\"ConnectorPlacement.EquallySpacedRectSide\",\"uuid\":\"43c1499b-0abd-4d60-8d0e-f99edfc99abb\"}]},\"type\":\"ConnectorPlacement.EquallySpacedConnector\",\"uuid\":\"7137f0d1-a693-433d-9f21-56f33280b1ef\"}],\"packageUris\":[\"http://schema.mathworks.com/mf0/Connector/R2020b\"],\"version\":\"1.0\"}"
  State selection : MATLAB Function  TreatAsAtomicUnit=on
  delta_v_a : Scope
  delta_x_a_3 : Scope
  s_i_a_3 : Scope
  u_I_a : Outport
  w_hat_a : Outport  Port=2
  wires:
  Angle controller/1(u_i_a) -> Scope/1, u_I_a/1
  Angle sliding variable/1(s_i_a) -> s_i_a_3/1, Angle controller/2(s_i_a)
  atti_ref/1 -> Sliding mode differentiator/1(Reference)
  states_i/1 -> State selection/1(states_i), Attitude loop observer/1(states_i)
  State selection/1(x_i_a) -> Attitude loop observer/2(x_i_a), Angle error/1(x_i_a)
  State selection/2(v_i_a) -> Attitude loop observer/3(v_i_a), Angle error/2(v_i_a)
  Sliding mode differentiator/3(ang_d) -> Angle error/3(ang_d)
  Angle error/1(delta_x_a) -> delta_x_a_3/1, Angle sliding variable/1(delta_x_a), Angle controller/3(delta_x_a)
  Angle error/2(delta_v_a) -> delta_v_a/1, Angle controller/4(delta_v_a), Angle sliding variable/2(delta_v_a)
  Attitude loop observer/2(w_hat_a) -> Angle controller/1(w_hat_a)
  Sliding mode differentiator/2(ang_d_ddot) -> Angle controller/5(ang_d_ddot)
  u_nom_a/1 -> Attitude loop observer/4(u_nom_a)
  Sliding mode differentiator/1(ang_d_dot) -> Angle error/4(ang_d_dot)
  Attitude loop observer/1(w_hat_a_actual) -> w_hat_a/1

== system Multi_drones_deri_and_intro_compare/Controller 3/Controller/Position controller1 ==
  states_i : Inport
  ref_x_p : Inport  Port=2
  u_nom_p : Inport  Port=3
  Constant : Constant  Value=[0;0;0]  VectorParams1D=off
  Error calculation : MATLAB Function  TreatAsAtomicUnit=on
  Position loop observer : Subsystem  mask{InitialCondition=[-2;4;0]}
      mask prompts: InitialCondition "Simulink:blkprm_prompts:IntegratorInitCond"
      settings: PortSchema="{\"entries\":[{\"content\":{\"sides\":[{\"content\":{\"connectorIds\":[\"In1\",\"In2\",\"In3\"]},\"type\":\"ConnectorPlacement.EquallySpacedRectSide\",\"uuid\":\"edf82c9f-eb15-4775-9311-d50d92fa47fd\"},{\"content\":{\"connectorIds\":[\"Out1\",\"Out2\"],\"side\":\"RIGHT\"},\"type\":\"ConnectorPlacement.EquallySpacedRectSide\",\"uuid\":\"b90416f6-8117-4ec7-8f9a-c5fae9711eab\"},{\"content\":{\"connectorIds\":[\"In4\"],\"side\":\"TOP\"},\"type\":\"ConnectorPlacement.EquallySpacedRectSide\",\"uuid\":\"e7e2e1a9-76d3-420a-917d-b73182cbe298\"}]},\"type\":\"ConnectorPlacement.EquallySpacedConnector\",\"uuid\":\"4fc8298e-c3da-4bdd-b1ba-c07bafbec956\"}],\"packageUris\":[\"http://schema.mathworks.com/mf0/Connector/R2020b\"],\"version\":\"1.0\"}"
      mask TypeOptions InitialCondition: x_int/InitialCondition
      mask DialogControl InitialCondition Prompt: Initial condition:
  Reference selection (Low) : MATLAB Function  TreatAsAtomicUnit=on
  State selection : MATLAB Function  TreatAsAtomicUnit=on
  Virtual position controller : MATLAB Function  TreatAsAtomicUnit=on
  delta_v_p_2 : Scope
  delta_x_p_3 : Scope
  s_i_p_3 : Scope
  u_i : Scope
  u_i_p : Outport
  w_hat_p : Outport  Port=2
  wires:
  states_i/1 -> Position loop observer/1(states_i), State selection/1(states_i)
  ref_x_p/1 -> Reference selection (Low)/1(ref_x_p)
  Reference selection (Low)/1(x_i_p_d) -> Error calculation/4(x_i_p_d)
  Reference selection (Low)/2(v_i_p_d) -> Error calculation/5(v_i_p_d)
  State selection/2(v_i_p) -> Position loop observer/3(v_i_p), Error calculation/2(v_i_p)
  State selection/1(x_i_p) -> Position loop observer/2(x_i_p), Error calculation/1(x_i_p)
  u_nom_p/1 -> Position loop observer/4(u_nom_p)
  Position loop observer/2(w_hat_p) -> Virtual position controller/1(w_hat_p)
  Reference selection (Low)/3(a_i_p_d) -> Virtual position controller/5(a_i_p_d)
  Constant/1 -> Error calculation/3(Phi_i)
  Error calculation/3(delta_v_p) -> delta_v_p_2/1, Virtual position controller/4(delta_v_p)
  Error calculation/2(delta_x_p) -> delta_x_p_3/1, Virtual position controller/3(delta_x_p)
  Error calculation/1(s_i_p) -> s_i_p_3/1, Virtual position controller/2(s_i_p)
  Virtual position controller/1(u_i_p) -> u_i_p/1, u_i/1
  Position loop observer/1(w_hat_p_actual) -> w_hat_p/1

== system Multi_drones_deri_and_intro_compare/Controller 3/Controller/Reverse calculation ==
  psi_id : Inport
  u_ip : Inport  Port=2
  states_i : Inport  Port=3
  Reverse calculation : MATLAB Function  TreatAsAtomicUnit=on
  State selection : MATLAB Function  TreatAsAtomicUnit=on
  atti_ref : Outport
  T_i_d : Outport  Port=2
  wires:
  Reverse calculation/2(T_i_d) -> T_i_d/1
  Reverse calculation/1(atti_ref) -> atti_ref/1
  states_i/1 -> State selection/1(states_i)
  State selection/1(x_i_a) -> Reverse calculation/3(x_i_a)
  u_ip/1 -> Reverse calculation/2(u_i_p)
  psi_id/1 -> Reverse calculation/1(psi_i_d)

== system Multi_drones_deri_and_intro_compare/Controller 4/Controller/Attitude controller ==
  states_i : Inport
  atti_ref : Inport  Port=2
  u_nom_a : Inport  Port=3
  Angle controller : MATLAB Function  TreatAsAtomicUnit=on
  Angle error : MATLAB Function  TreatAsAtomicUnit=on
  Angle sliding variable : MATLAB Function  TreatAsAtomicUnit=on
  Attitude loop observer : Subsystem
      settings: PortSchema="{\"entries\":[{\"content\":{\"sides\":[{\"content\":{\"connectorIds\":[\"In1\",\"In2\",\"In3\"]},\"type\":\"ConnectorPlacement.EquallySpacedRectSide\",\"uuid\":\"edf82c9f-eb15-4775-9311-d50d92fa47fd\"},{\"content\":{\"connectorIds\":[\"Out1\",\"Out2\"],\"side\":\"RIGHT\"},\"type\":\"ConnectorPlacement.EquallySpacedRectSide\",\"uuid\":\"b90416f6-8117-4ec7-8f9a-c5fae9711eab\"},{\"content\":{\"connectorIds\":[\"In4\"],\"side\":\"TOP\"},\"type\":\"ConnectorPlacement.EquallySpacedRectSide\",\"uuid\":\"e7e2e1a9-76d3-420a-917d-b73182cbe298\"}]},\"type\":\"ConnectorPlacement.EquallySpacedConnector\",\"uuid\":\"4fc8298e-c3da-4bdd-b1ba-c07bafbec956\"}],\"packageUris\":[\"http://schema.mathworks.com/mf0/Connector/R2020b\"],\"version\":\"1.0\"}"
  Scope : Scope
  Sliding mode differentiator : Subsystem
      settings: PortSchema="{\"entries\":[{\"content\":{\"sides\":[{\"content\":{\"connectorIds\":[\"In1\"]},\"type\":\"ConnectorPlacement.EquallySpacedRectSide\",\"uuid\":\"d0355641-aeac-4820-b7cd-f9621efbd127\"},{\"content\":{\"connectorIds\":[\"Out1\",\"Out2\"],\"side\":\"RIGHT\"},\"type\":\"ConnectorPlacement.EquallySpacedRectSide\",\"uuid\":\"185ec072-6206-4946-bebc-a6564ad10b6f\"},{\"content\":{\"connectorIds\":[\"Out3\"],\"side\":\"TOP\"},\"type\":\"ConnectorPlacement.EquallySpacedRectSide\",\"uuid\":\"43c1499b-0abd-4d60-8d0e-f99edfc99abb\"}]},\"type\":\"ConnectorPlacement.EquallySpacedConnector\",\"uuid\":\"7137f0d1-a693-433d-9f21-56f33280b1ef\"}],\"packageUris\":[\"http://schema.mathworks.com/mf0/Connector/R2020b\"],\"version\":\"1.0\"}"
  State selection : MATLAB Function  TreatAsAtomicUnit=on
  delta_v_a : Scope
  delta_x_a_4 : Scope
  s_i_a_4 : Scope
  u_I_a : Outport
  w_hat_a : Outport  Port=2
  wires:
  Angle controller/1(u_i_a) -> Scope/1, u_I_a/1
  Angle sliding variable/1(s_i_a) -> s_i_a_4/1, Angle controller/2(s_i_a)
  atti_ref/1 -> Sliding mode differentiator/1(Reference)
  states_i/1 -> State selection/1(states_i), Attitude loop observer/1(states_i)
  State selection/1(x_i_a) -> Attitude loop observer/2(x_i_a), Angle error/1(x_i_a)
  State selection/2(v_i_a) -> Attitude loop observer/3(v_i_a), Angle error/2(v_i_a)
  Sliding mode differentiator/3(ang_d) -> Angle error/3(ang_d)
  Angle error/1(delta_x_a) -> delta_x_a_4/1, Angle sliding variable/1(delta_x_a), Angle controller/3(delta_x_a)
  Angle error/2(delta_v_a) -> delta_v_a/1, Angle controller/4(delta_v_a), Angle sliding variable/2(delta_v_a)
  Attitude loop observer/2(w_hat_a) -> Angle controller/1(w_hat_a)
  Sliding mode differentiator/2(ang_d_ddot) -> Angle controller/5(ang_d_ddot)
  u_nom_a/1 -> Attitude loop observer/4(u_nom_a)
  Sliding mode differentiator/1(ang_d_dot) -> Angle error/4(ang_d_dot)
  Attitude loop observer/1(w_hat_a_actual) -> w_hat_a/1

== system Multi_drones_deri_and_intro_compare/Controller 4/Controller/Position controller1 ==
  states_i : Inport
  ref_x_p : Inport  Port=2
  u_nom_p : Inport  Port=3
  Constant : Constant  Value=[0;0;0]  VectorParams1D=off
  Error calculation : MATLAB Function  TreatAsAtomicUnit=on
  Position loop observer : Subsystem  mask{InitialCondition=[-4;-1;0]}
      mask prompts: InitialCondition "Simulink:blkprm_prompts:IntegratorInitCond"
      settings: PortSchema="{\"entries\":[{\"content\":{\"sides\":[{\"content\":{\"connectorIds\":[\"In1\",\"In2\",\"In3\"]},\"type\":\"ConnectorPlacement.EquallySpacedRectSide\",\"uuid\":\"edf82c9f-eb15-4775-9311-d50d92fa47fd\"},{\"content\":{\"connectorIds\":[\"Out1\",\"Out2\"],\"side\":\"RIGHT\"},\"type\":\"ConnectorPlacement.EquallySpacedRectSide\",\"uuid\":\"b90416f6-8117-4ec7-8f9a-c5fae9711eab\"},{\"content\":{\"connectorIds\":[\"In4\"],\"side\":\"TOP\"},\"type\":\"ConnectorPlacement.EquallySpacedRectSide\",\"uuid\":\"e7e2e1a9-76d3-420a-917d-b73182cbe298\"}]},\"type\":\"ConnectorPlacement.EquallySpacedConnector\",\"uuid\":\"4fc8298e-c3da-4bdd-b1ba-c07bafbec956\"}],\"packageUris\":[\"http://schema.mathworks.com/mf0/Connector/R2020b\"],\"version\":\"1.0\"}"
      mask TypeOptions InitialCondition: x_int/InitialCondition
      mask DialogControl InitialCondition Prompt: Initial condition:
  Reference selection (Low) : MATLAB Function  TreatAsAtomicUnit=on
  State selection : MATLAB Function  TreatAsAtomicUnit=on
  Virtual position controller : MATLAB Function  TreatAsAtomicUnit=on
  delta_v_p_4 : Scope
  delta_x_p_4 : Scope
  s_i_p_4 : Scope
  u_i : Scope
  u_i_p : Outport
  w_hat_p : Outport  Port=2
  wires:
  states_i/1 -> Position loop observer/1(states_i), State selection/1(states_i)
  ref_x_p/1 -> Reference selection (Low)/1(ref_x_p)
  Reference selection (Low)/1(x_i_p_d) -> Error calculation/4(x_i_p_d)
  Reference selection (Low)/2(v_i_p_d) -> Error calculation/5(v_i_p_d)
  State selection/2(v_i_p) -> Position loop observer/3(v_i_p), Error calculation/2(v_i_p)
  State selection/1(x_i_p) -> Position loop observer/2(x_i_p), Error calculation/1(x_i_p)
  u_nom_p/1 -> Position loop observer/4(u_nom_p)
  Position loop observer/2(w_hat_p) -> Virtual position controller/1(w_hat_p)
  Reference selection (Low)/3(a_i_p_d) -> Virtual position controller/5(a_i_p_d)
  Constant/1 -> Error calculation/3(Phi_i)
  Error calculation/3(delta_v_p) -> delta_v_p_4/1, Virtual position controller/4(delta_v_p)
  Error calculation/2(delta_x_p) -> delta_x_p_4/1, Virtual position controller/3(delta_x_p)
  Error calculation/1(s_i_p) -> s_i_p_4/1, Virtual position controller/2(s_i_p)
  Virtual position controller/1(u_i_p) -> u_i_p/1, u_i/1
  Position loop observer/1(w_hat_p_actual) -> w_hat_p/1

== system Multi_drones_deri_and_intro_compare/Controller 4/Controller/Reverse calculation ==
  psi_id : Inport
  u_ip : Inport  Port=2
  states_i : Inport  Port=3
  Reverse calculation : MATLAB Function  TreatAsAtomicUnit=on
  State selection : MATLAB Function  TreatAsAtomicUnit=on
  atti_ref : Outport
  T_i_d : Outport  Port=2
  wires:
  Reverse calculation/2(T_i_d) -> T_i_d/1
  Reverse calculation/1(atti_ref) -> atti_ref/1
  states_i/1 -> State selection/1(states_i)
  State selection/1(x_i_a) -> Reverse calculation/3(x_i_a)
  u_ip/1 -> Reverse calculation/2(u_i_p)
  psi_id/1 -> Reverse calculation/1(psi_i_d)

== system Multi_drones_deri_and_intro_compare/Controller 5/Controller/Attitude controller ==
  states_i : Inport
  atti_ref : Inport  Port=2
  u_nom_a : Inport  Port=3
  Angle controller : MATLAB Function  TreatAsAtomicUnit=on
  Angle error : MATLAB Function  TreatAsAtomicUnit=on
  Angle sliding variable : MATLAB Function  TreatAsAtomicUnit=on
  Attitude loop observer : Subsystem
      settings: PortSchema="{\"entries\":[{\"content\":{\"sides\":[{\"content\":{\"connectorIds\":[\"In1\",\"In2\",\"In3\"]},\"type\":\"ConnectorPlacement.EquallySpacedRectSide\",\"uuid\":\"edf82c9f-eb15-4775-9311-d50d92fa47fd\"},{\"content\":{\"connectorIds\":[\"Out1\",\"Out2\"],\"side\":\"RIGHT\"},\"type\":\"ConnectorPlacement.EquallySpacedRectSide\",\"uuid\":\"b90416f6-8117-4ec7-8f9a-c5fae9711eab\"},{\"content\":{\"connectorIds\":[\"In4\"],\"side\":\"TOP\"},\"type\":\"ConnectorPlacement.EquallySpacedRectSide\",\"uuid\":\"e7e2e1a9-76d3-420a-917d-b73182cbe298\"}]},\"type\":\"ConnectorPlacement.EquallySpacedConnector\",\"uuid\":\"4fc8298e-c3da-4bdd-b1ba-c07bafbec956\"}],\"packageUris\":[\"http://schema.mathworks.com/mf0/Connector/R2020b\"],\"version\":\"1.0\"}"
  Scope : Scope
  Sliding mode differentiator : Subsystem
      settings: PortSchema="{\"entries\":[{\"content\":{\"sides\":[{\"content\":{\"connectorIds\":[\"In1\"]},\"type\":\"ConnectorPlacement.EquallySpacedRectSide\",\"uuid\":\"d0355641-aeac-4820-b7cd-f9621efbd127\"},{\"content\":{\"connectorIds\":[\"Out1\",\"Out2\"],\"side\":\"RIGHT\"},\"type\":\"ConnectorPlacement.EquallySpacedRectSide\",\"uuid\":\"185ec072-6206-4946-bebc-a6564ad10b6f\"},{\"content\":{\"connectorIds\":[\"Out3\"],\"side\":\"TOP\"},\"type\":\"ConnectorPlacement.EquallySpacedRectSide\",\"uuid\":\"43c1499b-0abd-4d60-8d0e-f99edfc99abb\"}]},\"type\":\"ConnectorPlacement.EquallySpacedConnector\",\"uuid\":\"7137f0d1-a693-433d-9f21-56f33280b1ef\"}],\"packageUris\":[\"http://schema.mathworks.com/mf0/Connector/R2020b\"],\"version\":\"1.0\"}"
  State selection : MATLAB Function  TreatAsAtomicUnit=on
  delta_v_a_5 : Scope
  delta_x_a_5 : Scope
  s_i_a_5 : Scope
  u_I_a : Outport
  w_hat_a : Outport  Port=2
  wires:
  Angle controller/1(u_i_a) -> Scope/1, u_I_a/1
  Angle sliding variable/1(s_i_a) -> s_i_a_5/1, Angle controller/2(s_i_a)
  atti_ref/1 -> Sliding mode differentiator/1(Reference)
  states_i/1 -> State selection/1(states_i), Attitude loop observer/1(states_i)
  State selection/1(x_i_a) -> Attitude loop observer/2(x_i_a), Angle error/1(x_i_a)
  State selection/2(v_i_a) -> Attitude loop observer/3(v_i_a), Angle error/2(v_i_a)
  Sliding mode differentiator/3(ang_d) -> Angle error/3(ang_d)
  Angle error/1(delta_x_a) -> delta_x_a_5/1, Angle sliding variable/1(delta_x_a), Angle controller/3(delta_x_a)
  Angle error/2(delta_v_a) -> delta_v_a_5/1, Angle controller/4(delta_v_a), Angle sliding variable/2(delta_v_a)
  Attitude loop observer/2(w_hat_a) -> Angle controller/1(w_hat_a)
  Sliding mode differentiator/2(ang_d_ddot) -> Angle controller/5(ang_d_ddot)
  u_nom_a/1 -> Attitude loop observer/4(u_nom_a)
  Sliding mode differentiator/1(ang_d_dot) -> Angle error/4(ang_d_dot)
  Attitude loop observer/1(w_hat_a_actual) -> w_hat_a/1

== system Multi_drones_deri_and_intro_compare/Controller 5/Controller/Position controller1 ==
  states_i : Inport
  ref_x_p : Inport  Port=2
  u_nom_p : Inport  Port=3
  Constant : Constant  Value=[0;0;0]  VectorParams1D=off
  Error calculation : MATLAB Function  TreatAsAtomicUnit=on
  Position loop observer : Subsystem  mask{InitialCondition=[-1.5;-1;0]}
      mask prompts: InitialCondition "Simulink:blkprm_prompts:IntegratorInitCond"
      settings: PortSchema="{\"entries\":[{\"content\":{\"sides\":[{\"content\":{\"connectorIds\":[\"In1\",\"In2\",\"In3\"]},\"type\":\"ConnectorPlacement.EquallySpacedRectSide\",\"uuid\":\"edf82c9f-eb15-4775-9311-d50d92fa47fd\"},{\"content\":{\"connectorIds\":[\"Out1\",\"Out2\"],\"side\":\"RIGHT\"},\"type\":\"ConnectorPlacement.EquallySpacedRectSide\",\"uuid\":\"b90416f6-8117-4ec7-8f9a-c5fae9711eab\"},{\"content\":{\"connectorIds\":[\"In4\"],\"side\":\"TOP\"},\"type\":\"ConnectorPlacement.EquallySpacedRectSide\",\"uuid\":\"e7e2e1a9-76d3-420a-917d-b73182cbe298\"}]},\"type\":\"ConnectorPlacement.EquallySpacedConnector\",\"uuid\":\"4fc8298e-c3da-4bdd-b1ba-c07bafbec956\"}],\"packageUris\":[\"http://schema.mathworks.com/mf0/Connector/R2020b\"],\"version\":\"1.0\"}"
      mask TypeOptions InitialCondition: x_int/InitialCondition
      mask DialogControl InitialCondition Prompt: Initial condition:
  Reference selection (Low) : MATLAB Function  TreatAsAtomicUnit=on
  State selection : MATLAB Function  TreatAsAtomicUnit=on
  Virtual position controller : MATLAB Function  TreatAsAtomicUnit=on
  delta_v_p_5 : Scope
  delta_x_p_5 : Scope
  s_i_p_5 : Scope
  u_i : Scope
  u_i_p : Outport
  w_hat_p : Outport  Port=2
  wires:
  states_i/1 -> Position loop observer/1(states_i), State selection/1(states_i)
  ref_x_p/1 -> Reference selection (Low)/1(ref_x_p)
  Reference selection (Low)/1(x_i_p_d) -> Error calculation/4(x_i_p_d)
  Reference selection (Low)/2(v_i_p_d) -> Error calculation/5(v_i_p_d)
  State selection/2(v_i_p) -> Position loop observer/3(v_i_p), Error calculation/2(v_i_p)
  State selection/1(x_i_p) -> Position loop observer/2(x_i_p), Error calculation/1(x_i_p)
  u_nom_p/1 -> Position loop observer/4(u_nom_p)
  Position loop observer/2(w_hat_p) -> Virtual position controller/1(w_hat_p)
  Reference selection (Low)/3(a_i_p_d) -> Virtual position controller/5(a_i_p_d)
  Constant/1 -> Error calculation/3(Phi_i)
  Error calculation/3(delta_v_p) -> delta_v_p_5/1, Virtual position controller/4(delta_v_p)
  Error calculation/2(delta_x_p) -> delta_x_p_5/1, Virtual position controller/3(delta_x_p)
  Error calculation/1(s_i_p) -> s_i_p_5/1, Virtual position controller/2(s_i_p)
  Virtual position controller/1(u_i_p) -> u_i_p/1, u_i/1
  Position loop observer/1(w_hat_p_actual) -> w_hat_p/1

== system Multi_drones_deri_and_intro_compare/Controller 5/Controller/Reverse calculation ==
  psi_id : Inport
  u_ip : Inport  Port=2
  states_i : Inport  Port=3
  Reverse calculation : MATLAB Function  TreatAsAtomicUnit=on
  State selection : MATLAB Function  TreatAsAtomicUnit=on
  atti_ref : Outport
  T_i_d : Outport  Port=2
  wires:
  Reverse calculation/2(T_i_d) -> T_i_d/1
  Reverse calculation/1(atti_ref) -> atti_ref/1
  states_i/1 -> State selection/1(states_i)
  State selection/1(x_i_a) -> Reverse calculation/3(x_i_a)
  u_ip/1 -> Reverse calculation/2(u_i_p)
  psi_id/1 -> Reverse calculation/1(psi_i_d)
